simulink model "CRA_Assignment7"  (R2022b)
settings: Solver=VariableStepAuto  StartTime=0.0  StopTime=100  FixedStep=0.00001  RelTol=1e-3
libraries: simulink x1
settings Model: Creator=Andrea  LastModifiedBy=Andrea

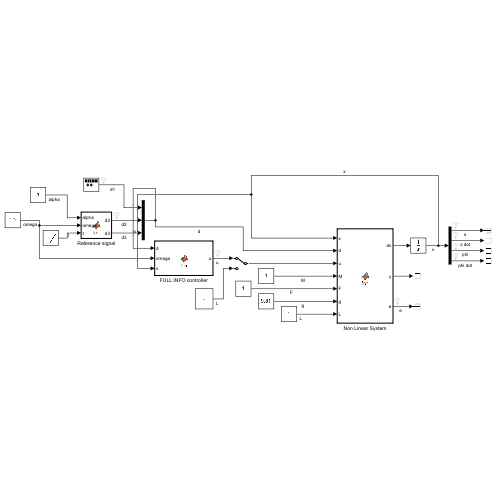
[thumbnail: Simulink's stored preview of the top-level diagram]
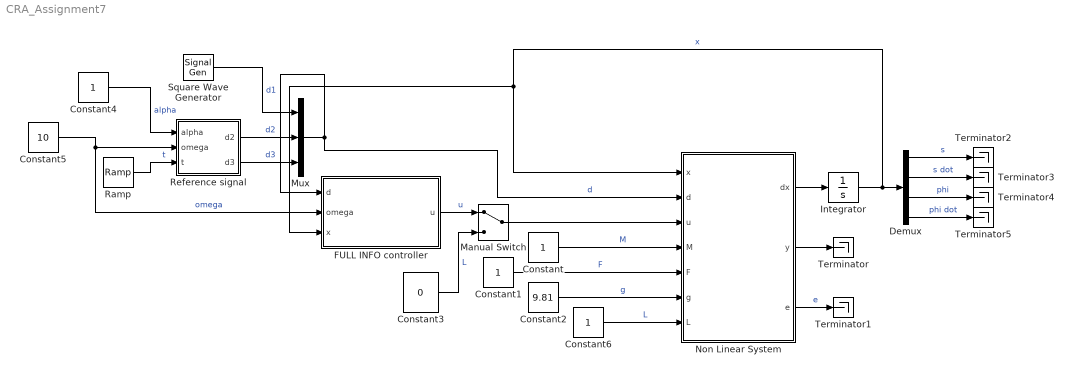
== system CRA_Assignment7 ==
  Constant{,1,4,6} (4 alike) : Constant
  Constant2 : Constant  Value=9.81
  Constant3 : Constant  Value=0
  Constant5 : Constant  Value=10
  Demux : Demux
  FULL INFO controller : MATLAB Function  TreatAsAtomicUnit=on
  Integrator : Integrator  InitialCondition=[0,0,0,0]  ContinuousStateAttributes='position_and_angle'
  Manual Switch : ManualSwitch
  Mux : Mux  Inputs=3
  Non Linear System : MATLAB Function  TreatAsAtomicUnit=on
  Ramp : simulink/Sources/Ramp  slope=1  start=0  InitialOutput=0
  Reference signal : MATLAB Function  TreatAsAtomicUnit=on
  Square Wave Generator : SignalGenerator  WaveForm=square  Amplitude=0.5  Frequency=0.02*2*3.16  Units=rad/sec
  Terminator{,1..5} (6 alike) : Terminator
  wires:
  Non Linear System/1(dx) -> Integrator/1
  Integrator/1 -> Non Linear System/1(x), FULL INFO controller/3(x), Demux/1  "x"
  Constant/1 -> Non Linear System/4(M)  "M"
  Constant1/1 -> Non Linear System/5(F)  "F"
  Constant2/1 -> Non Linear System/6(g)  "g"
  Mux/1 -> Non Linear System/2(d), FULL INFO controller/1(d)  "d"
  Square Wave Generator/1 -> Mux/1  "d1"
  Non Linear System/2(y) -> Terminator/1
  Non Linear System/3(e) -> Terminator1/1  "e"
  Reference signal/1(d2) -> Mux/2  "d2"
  Constant5/1 -> FULL INFO controller/2(omega), Reference signal/2(omega)  "omega"
  Constant4/1 -> Reference signal/1(alpha)  "alpha"
  Ramp/1 -> Reference signal/3(t)  "t"
  Constant6/1 -> Non Linear System/7(L)  "L"
  Reference signal/2(d3) -> Mux/3  "d3"
  Demux/1 -> Terminator2/1  "s"
  Demux/2 -> Terminator3/1  "s dot"
  Demux/3 -> Terminator4/1  "phi"
  Demux/4 -> Terminator5/1  "phi dot"
  FULL INFO controller/1(u) -> Manual Switch/1  "u"
  Manual Switch/1 -> Non Linear System/3(u)
  Constant3/1 -> Manual Switch/2  "L"

== matlab function CRA_Assignment7/FULL INFO controller ==
  data: d input; omega input; u output; x input
function u = fcn(d,omega,x)
% FULL INFO CONTROLLER  u=K*x+(Γ-K*Π)*d

Kx = 15.09683995922528*x(4)+47.25648318042813*x(3)+6.09683995922528*x(2)+2.446483180428134*x(1);
Ld = d(3)*((15.09683995922528*omega^3)/(omega^2+9.81)-5.09683995922528*omega)+d(2)*((47.25648318042813*omega^2)/(omega^2+9.81)-omega^2-2.446483180428134)-1.0*d(1);
u = Kx + Ld;

== matlab function CRA_Assignment7/Non Linear System ==
  data: x input; d input; dx output; u input; y output; M input; F input; g input; e output; L input
function [dx,y,e] = fcn(x,d,u,M,F,g,L)
dx = [0,0,0,0];
dx(1) = x (2);
dx(2) = -(x(2)*F-u-d(1))/M;
dx(3) = x(4);
dx(4) = (sin(x(3))*M*g+x(2)*cos(x(3))*F-u*cos(x(3))-d(1)*cos(x(3)))/(L*M);

y = [x(2), x(4)]';

e = d(2)-x(1);
end

== matlab function CRA_Assignment7/Reference signal ==
  data: alpha input; omega input; d2 output; t input; d3 output
function [d2,d3] = fcn(alpha,omega,t)
%#FULL INFO CONTROLLER  u=K*x+(Γ-K*Π)*d

d2 = alpha * sin(omega*t);
d3 = alpha * cos(omega*t);
end
